simulink model "shem3"  (R2023a)
settings: Solver=VariableStepAuto  StartTime=0.0  StopTime=10.0  RelTol=1e-3
settings Model: Creator=fynjy  LastModifiedBy=fynjy

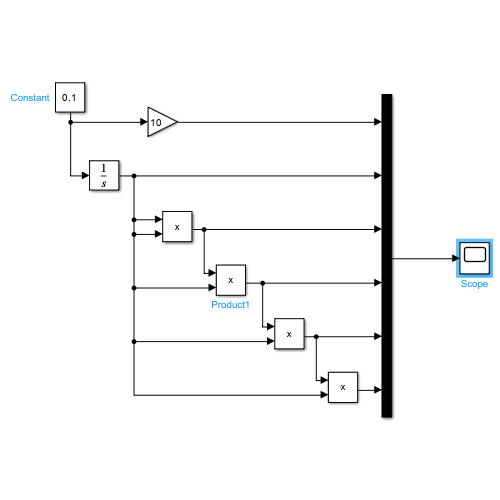
[thumbnail: Simulink's stored preview of the top-level diagram]
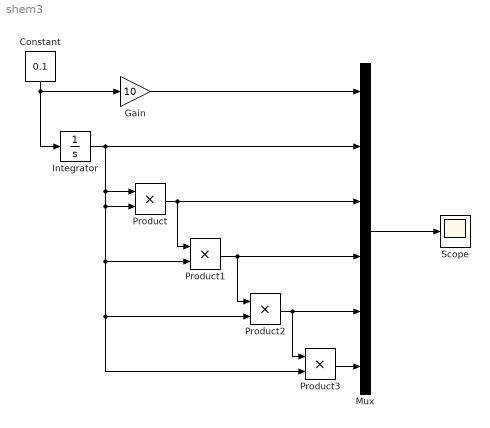
== system shem3 ==
  Constant : Constant  Value=0.1
  Gain : Gain  Gain=10
  Integrator : Integrator
  Mux : Mux  Inputs=6
  Product{,1..3} (4 alike) : Product
  Scope : Scope
  wires:
  Mux/1 -> Scope/1
  Constant/1 -> Gain/1, Integrator/1
  Gain/1 -> Mux/1
  Integrator/1 -> Product3/2, Product2/2, Product1/2, Product/2, Product/1, Mux/2
  Product/1 -> Product1/1, Mux/3
  Product1/1 -> Product2/1, Mux/4
  Product2/1 -> Product3/1, Mux/5
  Product3/1 -> Mux/6
